simulink model "HW13"  (R2025a)
settings: Solver=VariableStepAuto  StartTime=0.0  StopTime=10  RelTol=1e-3
undefined symbols (not defined in the file): Add, Fs, h, Shift
libraries: dspsrcs4 x1, dsphdlmathfun2 x1, dsphdlxfrm2 x1, dsphdlsigops2 x1
settings Model: Creator=gxoro  LastModifiedBy=gxoro

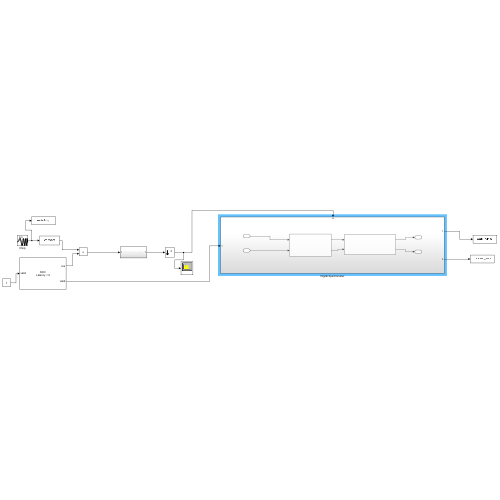
[thumbnail: Simulink's stored preview of the top-level diagram]
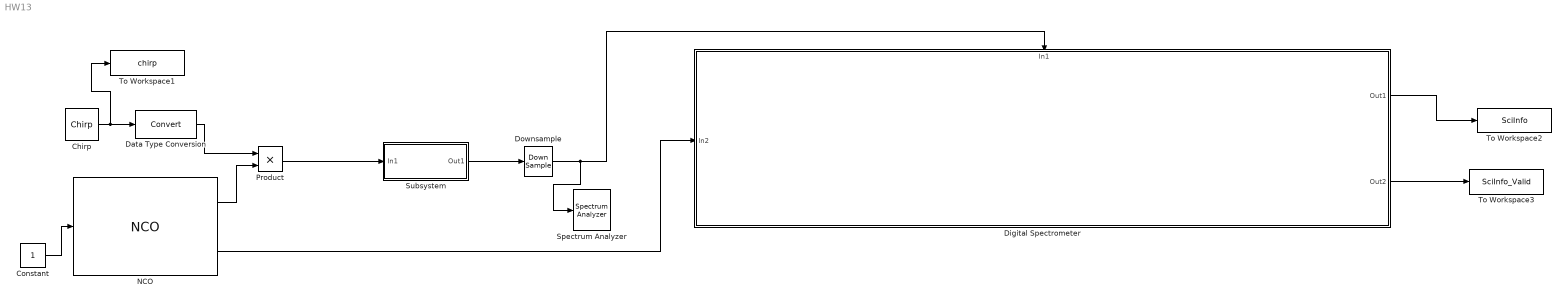
== system HW13 ==
  Chirp : dspsrcs4/Chirp  sweep=Linear  mode=Unidirectional  f0=10e6  f1=20e6  t1=0.00001998  Tsweep=0.00001998  phase=0  Ts=1/1/Fs  spf=1  datatype=double  OutputFrames=off
  Constant : Constant  OutDataTypeStr=boolean  SampleTime=1/Fs
  Data Type Conversion : DataTypeConversion  SaturateOnIntegerOverflow=off  RndMeth=Floor
  Digital Spectrometer : Subsystem
      settings: PortSchema="{\"entries\":[{\"content\":{\"sides\":[{\"content\":{\"connectorIds\":[\"In1\"]},\"type\":\"ConnectorPlacement.EquallySpacedRectSide\",\"uuid\":\"493d5d66-71f3-4239-bcd2-61c072bdca02\"},{\"content\":{\"connectorIds\":[\"Out1\",\"Out2\"],\"side\":\"RIGHT\"},\"type\":\"ConnectorPlacement.EquallySpacedRectSide\",\"uuid\":\"54bae7ff-46d4-4b56-9325-a0a1df53ad28\"},{\"content\":{\"connectorIds\":[\"In2\"],\"side\":\"TOP\"},\"type\":\"ConnectorPlacement.EquallySpacedRectSide\",\"uuid\":\"a6cfa3f0-f20a-4d18-9ba9-eff4c51790ec\"},{\"content\":{\"side\":\"BOTTOM\"},\"type\":\"ConnectorPlacement.EquallySpacedRectSide\",\"uuid\":\"f814c425-1a5a-47fa-84fd-540bcfd95cd8\"}]},\"type\":\"ConnectorPlacement.EquallySpacedConnector\",\"uuid\":\"dad7fa2f-9faf-414e-9186-d0c1bd135cb3\"}],\"packageUris\":[\"http://schema.mathworks.com/mf0/Connector/R2020b\"],\"version\":\"1.0\"}"
  Downsample : DownSample  AllowArbitraryFixedInput=on
  NCO : dsphdlsigops2/NCO  PhaseIncrementSource=Property  PhaseIncrement=phIncr  PhaseOffsetSource=Property  PhaseOffset=phOff  DitherSource=Property  NumDitherBits=dithBits  SamplesPerFrame=1  LUTCompress=off  ResetAction=off  Waveform=Cosine  PhasePort=off  SimulateUsing=Code generation  AccumulatorWL=N  PhaseQuantization=on  NumQuantizerAccumulatorBits=Q  OutputDataType=Binary point scaling  OutputWL=16  OutputFL=14
  Product : Product
  Spectrum Analyzer : SpectrumAnalyzer  WindowPosition=[560.000000,290.000000,800.000000,500.000000,]  ScopeFrameLocation=window  WindowInvariantSamplesPerUpdate=on  Span=60000000  StartFrequency=-30000000  StopFrequency=30000000  YLimits=[-78.4225 8.8722]
  Subsystem : Subsystem
  To Workspace1 : ToWorkspace  VariableName=chirp  SaveFormat=Timeseries  SampleTime=-1
  To Workspace2 : ToWorkspace  VariableName=SciInfo  SampleTime=-1
      settings: Save2DSignal=2-D array (concatenate along first dimension)
  To Workspace3 : ToWorkspace  VariableName=SciInfo_Valid  SampleTime=-1
      settings: Save2DSignal=2-D array (concatenate along first dimension)
  wires:
  Data Type Conversion/1 -> Product/1
  Constant/1 -> NCO/1
  Chirp/1 -> To Workspace1/1, Data Type Conversion/1
  Subsystem/1(Out1) -> Downsample/1
  NCO/1 -> Product/2
  Product/1 -> Subsystem/1(In1)
  Downsample/1 -> Spectrum Analyzer/1, Digital Spectrometer/2(In1)
  Digital Spectrometer/2(Out2) -> To Workspace3/1
  Digital Spectrometer/1(Out1) -> To Workspace2/1
  NCO/2 -> Digital Spectrometer/1(In2)

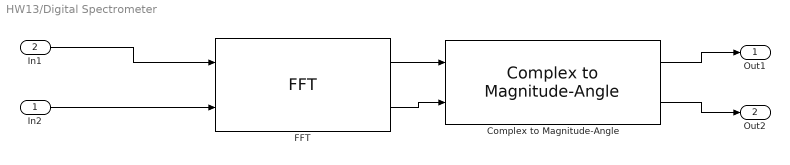
== system HW13/Digital Spectrometer ==
  In2 : Inport
  In1 : Inport  Port=2
  Complex to Magnitude-Angle : dsphdlmathfun2/Complex to Magnitude-Angle  NumIterationsSource=Auto  NumIterations=10  OutputFormat=Magnitude  AngleFormat=Normalized  ScaleOutput=on  ScalingMethod=Shift-Add  SimulateUsing=Code generation
  FFT : dsphdlxfrm2/FFT  Architecture=Streaming Radix 2^2  FFTLengthSource=Property  FFTLength=FFT  FFTLengthMax=1024  ComplexMultiplication=Use 4 multipliers and 2 adders  BitReversedOutput=off  BitReversedInput=off  Normalize=off  SimulateUsing=Code generation  RoundingMethod=Floor  ResetInputPort=off  StartOutputPort=off  EndOutputPort=off
  Out1 : Outport
  Out2 : Outport  Port=2
  wires:
  FFT/1 -> Complex to Magnitude-Angle/1
  Complex to Magnitude-Angle/2 -> Out2/1
  In1/1 -> FFT/1
  FFT/2 -> Complex to Magnitude-Angle/2
  Complex to Magnitude-Angle/1 -> Out1/1
  In2/1 -> FFT/2

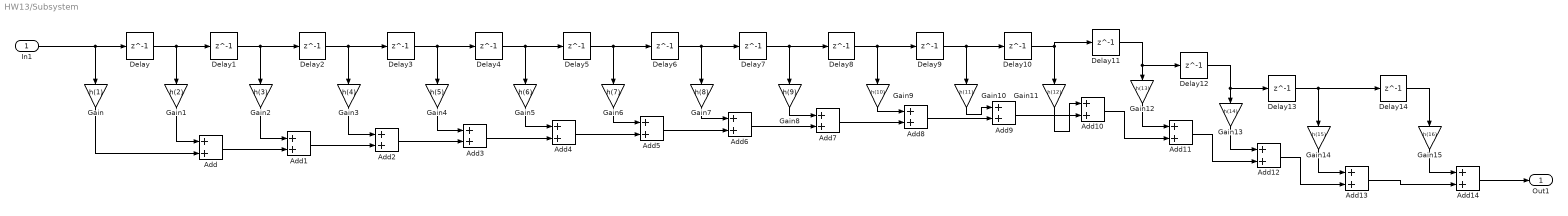
== system HW13/Subsystem ==
  In1 : Inport
  Add{,1..14} (15 alike) : Sum
  Delay{,1..14} (15 alike) : Delay  DelayLength=1  InitialCondition=0
  Gain : Gain  Gain=h(1)
  Gain1 : Gain  Gain=h(2)
  Gain10 : Gain  Gain=h(11)
  Gain11 : Gain  Gain=h(12)
  Gain12 : Gain  Gain=h(13)
  Gain13 : Gain  Gain=h(14)
  Gain14 : Gain  Gain=h(15)
  Gain15 : Gain  Gain=h(16)
  Gain2 : Gain  Gain=h(3)
  Gain3 : Gain  Gain=h(4)
  Gain4 : Gain  Gain=h(5)
  Gain5 : Gain  Gain=h(6)
  Gain6 : Gain  Gain=h(7)
  Gain7 : Gain  Gain=h(8)
  Gain8 : Gain  Gain=h(9)
  Gain9 : Gain  Gain=h(10)
  Out1 : Outport
  wires:
  In1/1 -> Delay/1, Gain/1
  Gain/1 -> Add/2
  Gain1/1 -> Add/1
  Delay/1 -> Delay1/1, Gain1/1
  Delay1/1 -> Gain2/1, Delay2/1
  Gain2/1 -> Add1/1
  Add/1 -> Add1/2
  Add1/1 -> Add2/2
  Gain3/1 -> Add2/1
  Delay2/1 -> Delay3/1, Gain3/1
  Add2/1 -> Add3/2
  Delay3/1 -> Delay4/1, Gain4/1
  Gain4/1 -> Add3/1
  Delay4/1 -> Delay5/1, Gain5/1
  Gain5/1 -> Add4/1
  Add3/1 -> Add4/2
  Delay5/1 -> Delay6/1, Gain6/1
  Gain6/1 -> Add5/1
  Add4/1 -> Add5/2
  Add5/1 -> Add6/2
  Delay6/1 -> Gain7/1, Delay7/1
  Gain7/1 -> Add6/1
  Add6/1 -> Add7/2
  Gain8/1 -> Add7/1
  Delay7/1 -> Delay8/1, Gain8/1
  Delay8/1 -> Delay9/1, Gain9/1
  Add7/1 -> Add8/2
  Gain9/1 -> Add8/1
  Gain10/1 -> Add9/1
  Delay9/1 -> Delay10/1, Gain10/1
  Add8/1 -> Add9/2
  Add9/1 -> Add10/2
  Delay10/1 -> Gain11/1, Delay11/1
  Gain11/1 -> Add10/1
  Gain12/1 -> Add11/1
  Add10/1 -> Add11/2
  Delay11/1 -> Delay12/1, Gain12/1
  Delay12/1 -> Delay13/1, Gain13/1
  Gain13/1 -> Add12/1
  Add11/1 -> Add12/2
  Delay13/1 -> Delay14/1, Gain14/1
  Add12/1 -> Add13/2
  Gain14/1 -> Add13/1
  Delay14/1 -> Gain15/1
  Add13/1 -> Add14/2
  Gain15/1 -> Add14/1
  Add14/1 -> Out1/1
